simulink model "HotPlateSISO_broida_reg"  (R2020b)
settings: Solver=VariableStepAuto  StartTime=0.0  StopTime=3600  RelTol=1e-3
undefined symbols (not defined in the file or in its folder): serial
libraries: instrumentlib x3, pid_lib x1
settings Model: Creator=busvelle  LastModifiedBy=Etudiants

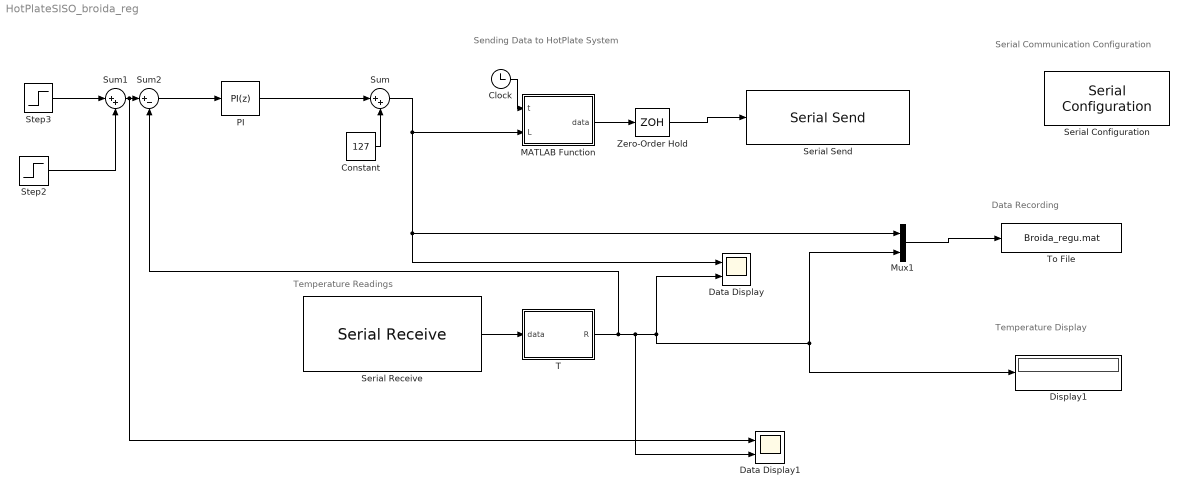
== system HotPlateSISO_broida_reg ==
  note: Data Recording
  note: Temperature Display
  note: Temperature Readings
  note: Serial Communication Configuration
  note: Sending Data to HotPlate System
  Clock : Clock
  Constant : Constant  Value=127
  Data Display : Scope  NumInputPorts=2
  Data Display1 : Scope  NumInputPorts=2
  Display1 : Display
  MATLAB Function : MATLAB Function  TreatAsAtomicUnit=on
  Mux1 : Mux  Inputs=2
  "PI " : pid_lib/PID Controller  Controller=PI  Form=Ideal  TimeDomain=Discrete-time  UseExternalTs=off  SampleTime=1  IntegratorMethod=Forward Euler  FilterMethod=Forward Euler  ControllerParametersSource=internal  P=5/0.148  I=1/330  D=0  UseFilter=on  N=100  TunerSelectOption=Transfer Function Based (PID Tuner App)  InitialConditionSource=internal  InitialConditionForIntegrator=0  InitialConditionForFilter=0  DifferentiatorICPrevScaledInput=0  ExternalReset=none  TrackingMode=off  Kt=1  LimitOutput=off  SatLimitsSource=internal  UpperSaturationLimit=inf  LowerSaturationLimit=-inf  LinearizeAsGain=off  AntiWindupMode=none  Kb=1  POutMin=[]  POutMax=[]  IOutMin=[]  IOutMax=[]  DOutMin=[]  DOutMax=[]  NOutMin=[]  NOutMax=[]  SumOutMin=[]  SumOutMax=[]  SaturationOutMin=[]  SaturationOutMax=[]  PParamMin=[]  PParamMax=[]  IParamMin=[]  IParamMax=[]  DParamMin=[]  DParamMax=[]  NParamMin=[]  NParamMax=[]  KbParamMin=[]  KbParamMax=[]  KtParamMin=[]  KtParamMax=[]  KbOutMin=[]  KbOutMax=[]  KtOutMin=[]  KtOutMax=[]  IntegratorOutMin=[]  IntegratorOutMax=[]  FilterOutMin=[]  FilterOutMax=[]  SumI1OutMin=[]  SumI1OutMax=[]  SumI2OutMin=[]  SumI2OutMax=[]  SumI3OutMin=[]  SumI3OutMax=[]  SumI4OutMin=[]  SumI4OutMax=[]  SumDOutMin=[]  SumDOutMax=[]  DifferentiatorOutMin=[]  DifferentiatorOutMax=[]  FilterDiffOutCoefMin=[]  FilterDiffOutCoefMax=[]  ReciprocalOutMin=[]  ReciprocalOutMax=[]  SumDenOutMin=[]  SumDenOutMax=[]  SumNumOutMin=[]  SumNumOutMax=[]  DivideOutMin=[]  DivideOutMax=[]  UdiffTsProdOutMin=[]  UdiffTsProdOutMax=[]  NTsProdOutMin=[]  NTsProdOutMax=[]  UintegralTsProdOutMin=[]  UintegralTsProdOutMax=[]  UngainTsProdOutMin=[]  UngainTsProdOutMax=[]  IntegratorContinuousStateAttributes=''  IntegratorStateMustResolveToSignalObject=off  IntegratorRTWStateStorageClass=Auto  FilterContinuousStateAttributes=''  FilterStateMustResolveToSignalObject=off  FilterRTWStateStorageClass=Auto  ParallelPVariant=Passthrough  IdealPVariant=InternalParameters  IVariant=InternalParameters  DVariant=Disabled  IntegratorVariant=Discrete  SatVariant=Disabled  AWVariant=Passthrough  PCopyVariant=Disabled  TRVariant=Disabled  FdbkBlocksVariant=Forward  IdealPFdbkVariant=Disabled  SatFdbkVariant=Disabled  DerivativeFilterVariant=Disabled  NVariant=Disabled  NCopyVariant=Disabled_SignalSpec  FilterICVariant=Disabled  IntegratorICVariant=InternalICs  ExternalResetVariant=Disabled  TRSumVariant=Passthrough  SumFdbkVariant=Disabled  SumVariant=Sum_PI  TsampFilterVariant=InternalTs  TsampNgainVariant=Passthrough  TsampIntegralVariant=Passthrough  ExternalSaturationOutDataTypeStr=Inherit: Same as second input
  Serial Configuration : instrumentlib/Serial Configuration  Priority=-200000  ComPortMenu=COM7  ComPort=COM7  ObjConstructor=serial('COM7');  BaudRate=9600  DataBits=8  Parity=none  StopBits=1  FlowControl=none  Timeout=2  ByteOrder=LittleEndian
  Serial Receive : instrumentlib/Serial Receive  ComPortMenu=COM7  ComPort=COM7  ObjConstructor=serial('COM7');  Terminator=<none>  DataSize="[1  9]"  DataType=uint8  EnableBlockingMode=on  ActionDataUnavailable=Output last received value  CustomValue=48+[0,2,3,0,0,0,2,3,0]  SampleTime=1
  Serial Send : instrumentlib/Serial Send  ComPortMenu=COM7  ComPort=COM7  ObjConstructor=serial('COM7');  Terminator=<none>  EnableBlockingMode=off
  Step2 : Step  Time=900  After=10  SampleTime=0
  Step3 : Step  Time=0  After=50  SampleTime=0
  Sum : Sum  Inputs=|++
  Sum1 : Sum  Inputs=|++
  Sum2 : Sum  Inputs=|+-
  T : MATLAB Function  TreatAsAtomicUnit=on
  To File : ToFile  Filename=Broida_regu.mat  MatrixName=data  SampleTime=1
  Zero-Order Hold : ZeroOrderHold
  wires:
  Serial Receive/1 -> T/1(data)
  Mux1/1 -> To File/1
  T/1(R) -> Sum2/2, Data Display1/2, Mux1/2, Display1/1, Data Display/2
  Zero-Order Hold/1 -> Serial Send/1
  MATLAB Function/1(data) -> Zero-Order Hold/1
  Clock/1 -> MATLAB Function/1(t)
  Sum/1 -> Data Display/1, Mux1/1, MATLAB Function/2(L)
  Step3/1 -> Sum1/1
  Step2/1 -> Sum1/2
  Sum1/1 -> Data Display1/1, Sum2/1
  Sum2/1 -> "PI "/1
  "PI "/1 -> Sum/1
  Constant/1 -> Sum/2

== matlab function HotPlateSISO_broida_reg/MATLAB Function ==
  data: t input; L input; data output
% function data = ToHotPlate(t,R,L)
function data = ToHotPlate(t,L)
if t<1
    fprintf('t=%7.2fs : Initialisation\n',t);
    data = uint8('D000980');% Base de temps
    pause(1);% le temps que l'Arduino commence à écouter...
elseif t>=3600*1.5
    fprintf('t=%7.2fs : RAZ\n',t);
    data = uint8('1000000');% RAZ
else
    L = min(max(0,round(L)),255);
    F = 0;
    R1 = 0; % mod(R,10);
    R2 = 0; %mod(R-R1,100)/10;
    R3 = 0; %(R-R1-10*R2)/100;
    L1 = mod(L,10);
    L2 = mod(L-L1,100)/10;
    L3 = (L-L1-10*L2)/100;
    data = uint8(48+[F,L3,L2,L1,R3,R2,R1]);
    if mod(t,60)==0
        fprintf('t=%7.2fs : U=(%5.1f,%5.1f)\n',t,0,L);
    end
end

== matlab function HotPlateSISO_broida_reg/T ==
  data: data input; R output
function R = FromHotPlate(data)
y = double(data-48);
% L = (y(1)*10+y(2))*10+y(3)+y(4)/10;
R = (y(6)*10+y(7))*10+y(8)+y(9)/10;
